simulink model "sin_compensar_discreto_potenciometro"  (R2015a)
settings: Solver=ode45  StartTime=0.0  StopTime=30  RelTol=1e-3
undefined symbols (not defined in the file): Bm, DisAng, Ga, Gb, Jt, Kb, Ki, L, Objetivo, PosInicial, Potenciometro, R, RelacionEngranajes, Rrueda
settings Model: Creator=familia colazo  LastModifiedBy=familia colazo

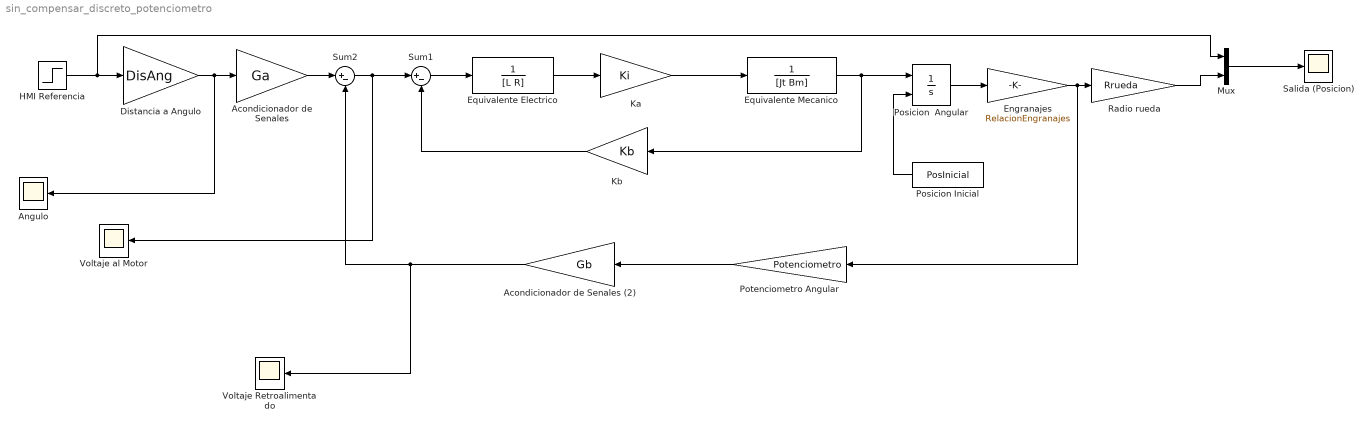
== system sin_compensar_discreto_potenciometro ==
  "Acondicionador de Senales " : Gain  Gain=Ga
  "Acondicionador de Senales (2) " : Gain  Gain=Gb
  Angulo : Scope
      settings: TickLabels=on  TimeRange=14  YMin=-0.751036  YMax=0.0612263  SaveName=ScopeData3  SampleInput=on
  "Distancia a Angulo " : Gain  Gain=DisAng
  "Engranajes " : Gain  Gain=RelacionEngranajes
  Equivalente Electrico : TransferFcn  Denominator=[L R]
  Equivalente Mecanico : TransferFcn  Denominator=[Jt Bm]
  HMI Referencia : Step  Time=0  After=Objetivo  SampleTime=0
  Ka : Gain  Gain=Ki
  Kb : Gain  Gain=Kb
  Mux : Mux  Inputs=2
  Posicion  Angular : Integrator  InitialConditionSource=external
  Posicion Inicial : Constant  Value=PosInicial
  "Potenciometro Angular " : Gain  Gain=Potenciometro
  Radio rueda : Gain  Gain=Rrueda
  Salida (Posicion) : Scope
      settings: TickLabels=on  TimeRange=14  YMin=-0.751036  YMax=0.0612263  SampleInput=on
  Sum1 : Sum  Inputs=|+-
  Sum2 : Sum  Inputs=|+-
  Voltaje Retroalimentado : Scope
      settings: TickLabels=on  TimeRange=14  YMin=-0.751036  YMax=0.0612263  SampleInput=on
  Voltaje al Motor : Scope
      settings: TickLabels=on  TimeRange=14  YMin=-0.751036  YMax=0.0612263  SaveName=ScopeData2  SampleInput=on
  wires:
  Mux/1 -> Salida (Posicion)/1
  HMI Referencia/1 -> Mux/1, "Distancia a Angulo "/1
  "Acondicionador de Senales (2) "/1 -> Voltaje Retroalimentado/1, Sum2/2
  Posicion Inicial/1 -> Posicion  Angular/2
  Sum2/1 -> Sum1/1, Voltaje al Motor/1
  Kb/1 -> Sum1/2
  Equivalente Mecanico/1 -> Kb/1, Posicion  Angular/1
  Equivalente Electrico/1 -> Ka/1
  Sum1/1 -> Equivalente Electrico/1
  Ka/1 -> Equivalente Mecanico/1
  "Engranajes "/1 -> "Potenciometro Angular "/1, Radio rueda/1
  "Acondicionador de Senales "/1 -> Sum2/1
  Radio rueda/1 -> Mux/2
  Posicion  Angular/1 -> "Engranajes "/1
  "Potenciometro Angular "/1 -> "Acondicionador de Senales (2) "/1
  "Distancia a Angulo "/1 -> Angulo/1, "Acondicionador de Senales "/1
